simulink model "zadatak1"  (Simulink 8.8)
settings: Solver=VariableStepAuto  StartTime=0.0  StopTime=300  RelTol=1e-3
values from neighbouring files (symbols this model uses):
  Kp = (1-exp(-T/Ts))/K0/(exp(T/T0) - 1)/(1 + N*(1 - exp(-T/Ts)))    [Parametri.m]
  T = 1    [Parametri.m]
undefined symbols (not defined in the file or in its folder): Td, Ti
libraries: simulink x1
settings Model: SuppressorTable="22 serialization::archive 11 0 6 0 0 1 8 0 0 0 0 6 0 0 1 0 48 zadatak1/Repeating Sequence Stair/LimitedCounter 0 6 0 0 2 8 0 0 0 0 6 41 Simulink:DataType:WarningOverFlowDetected 0 0 0 6 0  0  0 0 0 0 8 20160608 0 0 0 15 23 17 0 1 40 SimulinkFixedPoint:util:Overflowoccurred 0 0 0  0  8 20160608 0 15 23 17 0 1"  Creator=User  LastModifiedBy=User
settings DataIOCC: LimitDataPoints=off  SaveFormat=Dataset  SignalLoggingSaveFormat=Dataset
settings OptimizationCC: LifeSpan=auto
settings DebuggingCC: UnderspecifiedInitializationDetection=Simplified  MergeDetectMultiDrivingBlocksExec=error  FcnCallInpInsideContextMsg=error  StateNameClashWarn=none  SFUnexpectedBacktrackingDiag=error  SFNoUnconditionalDefaultTransitionDiag=error  SFExecutionAtInitializationDiag=warning
settings HardwareCC: ProdBitPerPointer=64  ProdBitPerSizeT=64  ProdBitPerPtrDiffT=64  ProdLargestAtomicFloat=Float  ProdIntDivRoundTo=Zero  ProdEndianess=LittleEndian  ProdWordSize=64  ProdHWDeviceType=Intel->x86-64 (Windows64)
settings ModelReferenceCC: PropagateSignalLabelsOutOfModel=on
settings GRTTargetCC: TargetLangStandard=C99 (ISO)  GeneratePreprocessorConditionals=Use local settings  CombineOutputUpdateFcns=on  GRTInterface=off
settings ConfigComp: CovMetricSettings=dwe  CovHtmlReporting=off  CovSaveCumulativeToWorkspaceVar=off  CovSaveSingleToWorkspaceVar=off  CovExternalEMLEnable=on

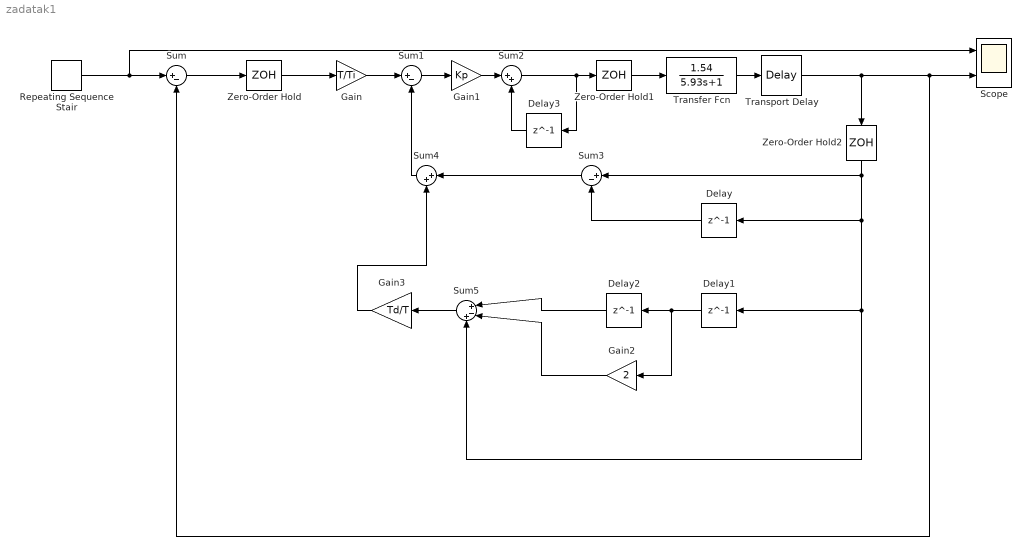
== system zadatak1 ==
  Delay{,1..3} (4 alike) : Delay  DelayLength=1
  Gain : Gain  Gain=T/Ti
  Gain1 : Gain  Gain=Kp
  Gain2 : Gain  Gain=2
  Gain3 : Gain  Gain=Td/T
  Repeating Sequence Stair : simulink/Sources/Repeating Sequence Stair  OutValues=[3 1 -5 2 1].'  tsamp=50  OutMin=[]  OutMax=[]  OutDataTypeStr=double  OutputDataTypeScalingMode=double  OutDataType=fixdt(0,8)  ConRadixGroup=Best Precision: Vector-wise  OutScaling=2^-12
  Scope : Scope  NumInputPorts=2
  Sum : Sum  Inputs=|+-
  Sum1 : Sum  Inputs=|+-
  Sum2 : Sum  Inputs=|++
  Sum3 : Sum  Inputs=|+-
  Sum4 : Sum  Inputs=|++
  Sum5 : Sum  Inputs=|+-+
  Transfer Fcn : TransferFcn  Numerator=[1.54]  Denominator=[5.93 1]
  Transport Delay : TransportDelay  DelayTime=1.07
  Zero-Order Hold : ZeroOrderHold  SampleTime=T
  Zero-Order Hold1 : ZeroOrderHold  SampleTime=T
  Zero-Order Hold2 : ZeroOrderHold  SampleTime=T
  wires:
  Repeating Sequence Stair/1 -> Scope/1, Sum/1
  Sum/1 -> Zero-Order Hold/1
  Zero-Order Hold/1 -> Gain/1
  Gain/1 -> Sum1/1
  Sum1/1 -> Gain1/1
  Gain1/1 -> Sum2/1
  Sum2/1 -> Delay3/1, Zero-Order Hold1/1
  Zero-Order Hold1/1 -> Transfer Fcn/1
  Transfer Fcn/1 -> Transport Delay/1
  Delay/1 -> Sum3/2
  Sum3/1 -> Sum4/1
  Delay1/1 -> Gain2/1, Delay2/1
  Delay2/1 -> Sum5/1
  Gain2/1 -> Sum5/2
  Zero-Order Hold2/1 -> Sum5/3, Delay1/1, Delay/1, Sum3/1
  Delay3/1 -> Sum2/2
  Sum5/1 -> Gain3/1
  Gain3/1 -> Sum4/2
  Sum4/1 -> Sum1/2
  Transport Delay/1 -> Sum/2, Scope/2, Zero-Order Hold2/1
